simulink model "MPC_Design"  (R2017a)
settings: Solver=VariableStepAuto  StartTime=0.0  StopTime=.3  MaxStep=1e-4  RelTol=1e-3
undefined symbols (not defined in the file or in its folder): G, GF
settings Model: Creator=erich  LastModifiedBy=erich

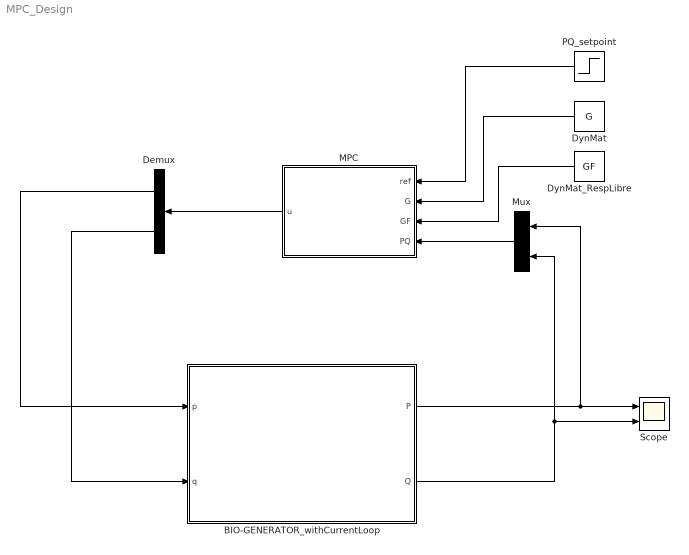
== system MPC_Design ==
  BIO-GENERATOR_withCurrentLoop : Subsystem
  Demux : Demux  Outputs=2
  DynMat : Constant  Value=G
  DynMat_RespLibre : Constant  Value=GF
  MPC : MATLAB Function  TreatAsAtomicUnit=on
  Mux : Mux  Inputs=2
  PQ_setpoint : Step  Time=[.1 .2]  Before=[0 0]  After=[500 2500]  SampleTime=0
  Scope : Scope  NumInputPorts=2
  wires:
  BIO-GENERATOR_withCurrentLoop/2(Q) -> Mux/2, Scope/2
  BIO-GENERATOR_withCurrentLoop/1(P) -> Mux/1, Scope/1
  DynMat_RespLibre/1 -> MPC/3(GF)
  DynMat/1 -> MPC/2(G)
  Mux/1 -> MPC/4(PQ)
  PQ_setpoint/1 -> MPC/1(ref)
  MPC/1(u) -> Demux/1
  Demux/1 -> BIO-GENERATOR_withCurrentLoop/1(p)
  Demux/2 -> BIO-GENERATOR_withCurrentLoop/2(" q")

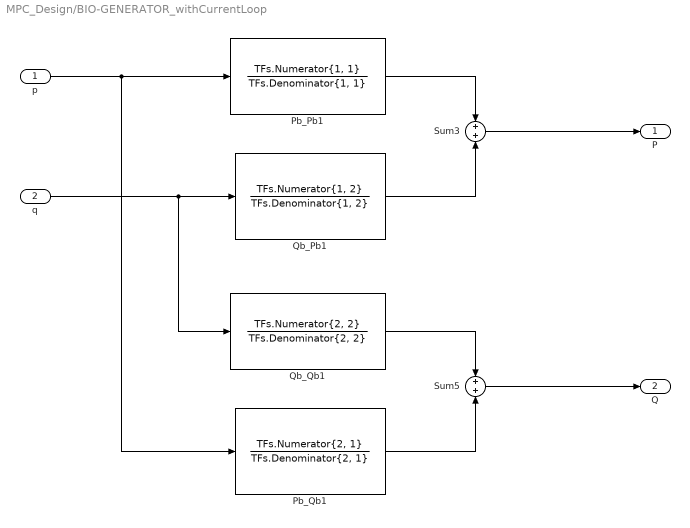
== system MPC_Design/BIO-GENERATOR_withCurrentLoop ==
  p : Inport
  " q" : Inport  Port=2
  Pb_Pb1 : TransferFcn  Numerator=TFs.Numerator{1, 1}  Denominator=TFs.Denominator{1, 1}
  Pb_Qb1 : TransferFcn  Numerator=TFs.Numerator{2, 1}  Denominator=TFs.Denominator{2, 1}
  Qb_Pb1 : TransferFcn  Numerator=TFs.Numerator{1, 2}  Denominator=TFs.Denominator{1, 2}
  Qb_Qb1 : TransferFcn  Numerator=TFs.Numerator{2, 2}  Denominator=TFs.Denominator{2, 2}
  Sum3 : Sum  Inputs=+|+
  Sum5 : Sum  Inputs=+|+
  P : Outport
  Q : Outport  Port=2
  wires:
  Qb_Pb1/1 -> Sum3/2
  Pb_Pb1/1 -> Sum3/1
  p/1 -> Pb_Pb1/1, Pb_Qb1/1
  Sum5/1 -> Q/1
  Pb_Qb1/1 -> Sum5/2
  Sum3/1 -> P/1
  Qb_Qb1/1 -> Sum5/1
  " q"/1 -> Qb_Pb1/1, Qb_Qb1/1

== matlab function MPC_Design/MPC ==
  data: ref input; G input; u output; GF input; PQ input
function u = MPC_DMC(ref, G, GF, PQ)


%%parametros del MPC
lamb = [1 .01]; % pesos de la funcion de coste J
p = 30; % horizonte de prediccion
nc = 10; % horizonte de control
N = 345; % tamaño de la respuesta al modelo del escalon

%% variables del MPC
persistent Du; % deltas de u 
persistent out; % salida actual del conrolador MPC.
persistent D; % matriz de diferencias;

if isempty(Du) % inicializacion de los deltas de uu
    Du = zeros(2*N, 1);
end

if isempty(out) % inicializaion de la salida del controlador MPC
    out = [0; 0];
end

if isempty(D) % inicializaion de la salida del controlador MPC
    z = zeros();
    D = [0; 0];
end


%% Calculo de la salida de control.

[G GF] = DMGen(Kcal, Tcal, Kenf, Tenf, Ts, N, p, nc);% obtencion DMC

H = G'*G*lamb(1)+lamb(1)*lamb(2)*eye(nc); % parte cuadratica del qp

ym = ones(p, 1)*T; % vector de la medida de tempearatura actual.

w = ones(p, 1)*ref; % vector señal setpoint.

L = GF*Du+ym; % respuesta libre.

F = 2*lamb(1)*(L-w)'*G; % parte lineal del problema qp.

duv = qpSimp(H, F', opt); % se soluciona J, se hallan los nc deltas de u optimos.

du = [duv(1), duv(6)]; % se extrae el primer du de calentador y primer du de enfriador

du = limsimp(0, 5, out, du); % se aplica la restriccion de la salida de 0 - 5 V.

Du = [du(1); Du(1:N-1); du(2); Du(N+1:end-1)];% actualizar historial deltas de u.

out = [ out(1)+du(1); out(2)+du(2) ]; %calcular salida del controlador.

ua = out;


u = 1;
